simulink model "SWC_AFE_Control"  (R2022b)
settings: configuration reference "DC_DC_Charger_Configuration" (kept outside this file)
undefined symbols (not defined in the file or in its folder): DUTY_COUNT_LOWER_LMIT, DUTY_COUNT_UPPER_LMIT, Fault_Counts_perms, GRID_NORM_FREQ, GRID_VOLT_ADC_OFFSET, HALF_DUTY_PERIOD, INDUCTANCE, PI, PLL_FREQ_LOW_LIMIT, PLL_FREQ_UPP_LIMIT, PLL_PI_INTGRL_RESET, PLL_PI_KI, PLL_PI_KP, PLL_PI_LOWER_LIMIT, PLL_PI_UPPER_LIMIT, PLL_RATE, PLL_VD_ERROR_LIMIT, PLL_VD_ESTIMETED, PLL_VQ_ERROR_LIMIT, VDC_LOWER_LIM_SVPWM, VDC_UPPER_LIM_SVPWM
libraries: simulink x13, common_lib x8
(part 1 of 2)
settings Model: DataDictionary=SWC_Diag_AFE.sldd  ExtModeTrigDuration=8  Creator=E0654638  LastModifiedBy=E0660158
settings ConfigSetRef: SourceName=DC_DC_Charger_Configuration

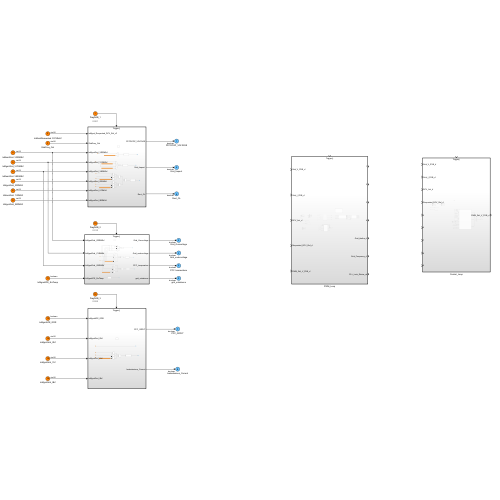
[thumbnail: Simulink's stored preview of the top-level diagram]
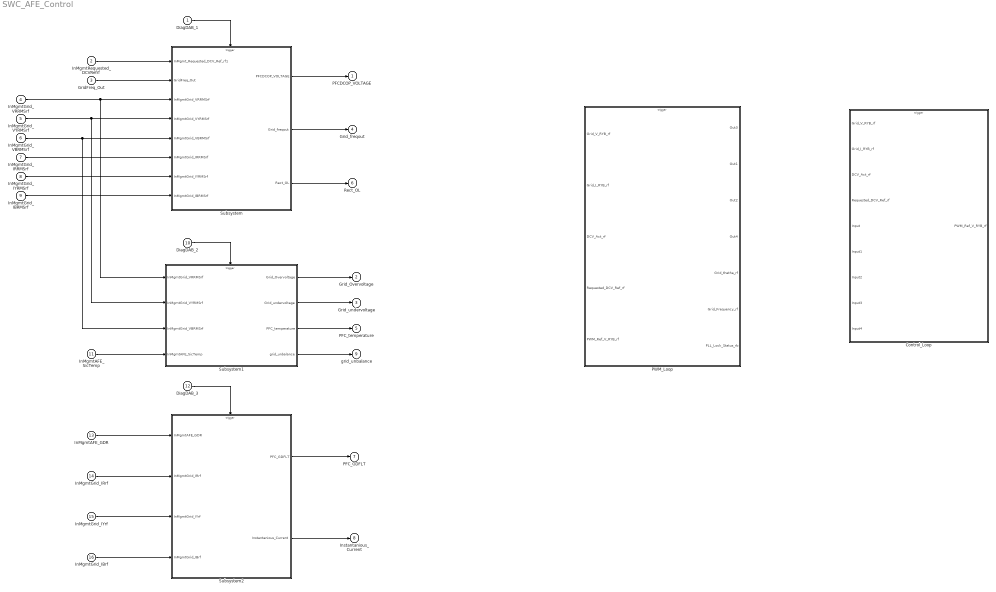
== system SWC_AFE_Control ==
  DiagDAB_1 : Inport  Description=Inverter HVDC voltage  OutMin=0  OutMax=1000  PortDimensions=1  SampleTime=0.001  OutputFunctionCall=on
      settings: AttributesFormatString=%<SampleTime>
  InMgmtRequested_DCVRefrf : Inport  Port=2  OutDataTypeStr=uint16
  GridFreq_Out : Inport  Port=3  OutDataTypeStr=uint16
  InMgmtGrid_VRRMSrf : Inport  Port=4  OutDataTypeStr=uint16
  InMgmtGrid_VYRMSrf : Inport  Port=5  OutDataTypeStr=uint16
  InMgmtGrid_VBRMSrf : Inport  Port=6  OutDataTypeStr=uint16
  InMgmtGrid_IRRMSrf : Inport  Port=7  OutDataTypeStr=uint16
  InMgmtGrid_IYRMSrf : Inport  Port=8  OutDataTypeStr=uint16
  InMgmtGrid_IBRMSrf : Inport  Port=9  OutDataTypeStr=uint16
  DiagDAB_2 : Inport  Description=Inverter HVDC voltage  Port=10  OutMin=0  OutMax=1000  PortDimensions=1  SampleTime=0.010  OutputFunctionCall=on
      settings: AttributesFormatString=%<SampleTime>
  InMgmtAFE_SicTemp : Inport  Port=11  OutDataTypeStr=boolean
  DiagDAB_3 : Inport  Description=Inverter HVDC voltage  Port=12  OutMin=0  OutMax=1000  PortDimensions=1  SampleTime=0.025  OutputFunctionCall=on
      settings: AttributesFormatString=%<SampleTime>
  InMgmtAFE_GDR : Inport  Port=13  OutDataTypeStr=boolean
  InMgmtGrid_IRrf : Inport  Port=14  OutDataTypeStr=uint16
  InMgmtGrid_IYrf : Inport  Port=15  OutDataTypeStr=uint16
  InMgmtGrid_IBrf : Inport  Port=16  OutDataTypeStr=uint16
  Control_Loop : Subsystem  Description=|  TreatAsAtomicUnit=on
      | @file      Control_Loop
      | @brief    All control related functions
      | @param[in]  required signals
      | @param[out] xxxxx
      | @return     None
      | @date       20/01/2023
      | @author     PKS (E0732241) @praveenksingh2@eaton.com
      | @copyright  Chief Engineer's office-EIIC
      settings: RTWSystemCode=Nonreusable function  RTWFcnNameOpts=Use subsystem name  RTWFileNameOpts=Use subsystem name
  PWM_Loop : Subsystem  Description=|  TreatAsAtomicUnit=on
      | @file       PWM_Loop
      | @brief      All algo related to PWM Control
      | @param[in]  required signals
      | @param[out] Duty values
      | @return     None
      | @date       20/01/2023
      | @author     PKS (E0732241) @praveenksingh2@eaton.com
      | @copyright  Chief Engineer's office-EIIC
      settings: RTWSystemCode=Nonreusable function  RTWFcnNameOpts=Use subsystem name  RTWFileNameOpts=Use subsystem name
  Subsystem : Subsystem
  Subsystem1 : Subsystem
  Subsystem2 : Subsystem
  PFCDCOP_VOLTAGE : Outport  OutDataTypeStr=boolean  VectorParamsAs1DForOutWhenUnconnected=off
  Grid_Overvoltage : Outport  Port=2  OutDataTypeStr=boolean  VectorParamsAs1DForOutWhenUnconnected=off
  Grid_undervoltage : Outport  Port=3  OutDataTypeStr=boolean  VectorParamsAs1DForOutWhenUnconnected=off
  "Grid_freqout " : Outport  Port=4  OutDataTypeStr=boolean  VectorParamsAs1DForOutWhenUnconnected=off
  PFC_temperature : Outport  Port=5  OutDataTypeStr=boolean  VectorParamsAs1DForOutWhenUnconnected=off
  Rect_OL : Outport  Port=6  OutDataTypeStr=boolean  VectorParamsAs1DForOutWhenUnconnected=off
  PFC_GDFLT : Outport  Port=7  OutDataTypeStr=boolean  VectorParamsAs1DForOutWhenUnconnected=off
  Instantanious_Current : Outport  Port=8  OutDataTypeStr=boolean  VectorParamsAs1DForOutWhenUnconnected=off
  grid_unbalance : Outport  Port=9  OutDataTypeStr=boolean  VectorParamsAs1DForOutWhenUnconnected=off
  wires:
  InMgmtRequested_DCVRefrf/1 -> Subsystem/1(InMgmt_Requested_DCV_Ref_rf1)
  Subsystem/1(PFCDCOP_VOLTAGE) -> PFCDCOP_VOLTAGE/1
  DiagDAB_1/1 -> Subsystem/Trigger
  InMgmtGrid_VRRMSrf/1 -> Subsystem1/1(InMgmtGrid_VRRMSrf), Subsystem/3(InMgmtGrid_VRRMSrf)
  InMgmtGrid_VYRMSrf/1 -> Subsystem1/2(InMgmtGrid_VYRMSrf), Subsystem/4(InMgmtGrid_VYRMSrf)
  InMgmtGrid_VBRMSrf/1 -> Subsystem1/3(InMgmtGrid_VBRMSrf), Subsystem/5(InMgmtGrid_VBRMSrf)
  Subsystem1/1(Grid_Overvoltage) -> Grid_Overvoltage/1
  DiagDAB_2/1 -> Subsystem1/Trigger
  Subsystem1/2(Grid_undervoltage) -> Grid_undervoltage/1
  GridFreq_Out/1 -> Subsystem/2(GridFreq_Out)
  Subsystem/2("Grid_freqout ") -> "Grid_freqout "/1
  InMgmtAFE_SicTemp/1 -> Subsystem1/4(InMgmtAFE_SicTemp)
  Subsystem1/3(PFC_temperature) -> PFC_temperature/1
  Subsystem/3(Rect_OL) -> Rect_OL/1
  Subsystem2/2(Instantanious_Current) -> Instantanious_Current/1
  InMgmtGrid_IBRMSrf/1 -> Subsystem/8(InMgmtGrid_IBRMSrf)
  InMgmtGrid_IYRMSrf/1 -> Subsystem/7(InMgmtGrid_IYRMSrf)
  InMgmtGrid_IRRMSrf/1 -> Subsystem/6(InMgmtGrid_IRRMSrf)
  DiagDAB_3/1 -> Subsystem2/Trigger
  Subsystem2/1(PFC_GDFLT) -> PFC_GDFLT/1
  InMgmtAFE_GDR/1 -> Subsystem2/1(InMgmtAFE_GDR)
  Subsystem1/4(grid_unbalance) -> grid_unbalance/1
  InMgmtGrid_IRrf/1 -> Subsystem2/2(InMgmtGrid_IRrf)
  InMgmtGrid_IYrf/1 -> Subsystem2/3(InMgmtGrid_IYrf)
  InMgmtGrid_IBrf/1 -> Subsystem2/4(InMgmtGrid_IBrf)

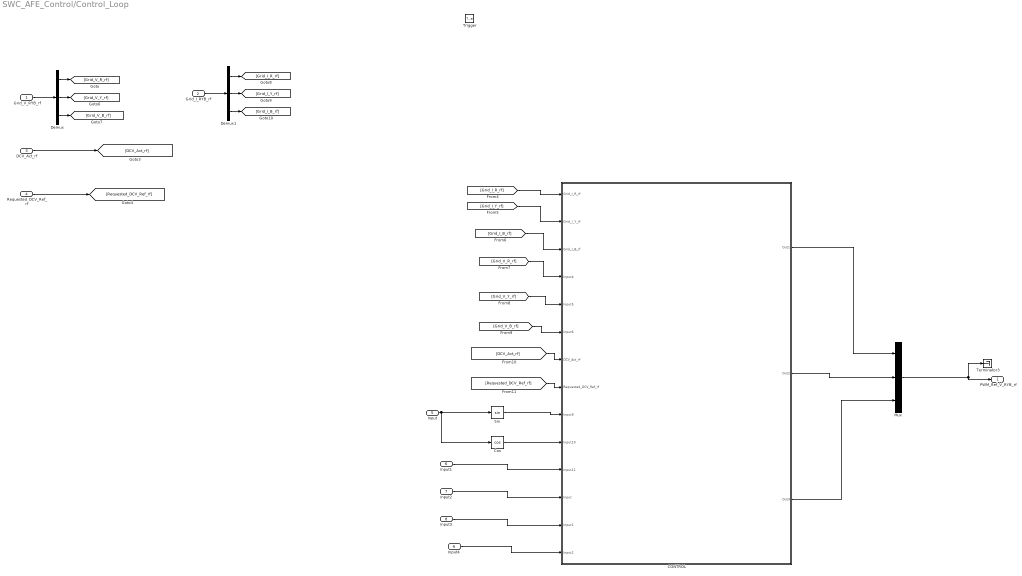
== system SWC_AFE_Control/Control_Loop ==
  Grid_V_RYB_rf : Inport
  Grid_I_RYB_rf : Inport  Port=2
  DCV_Act_rf : Inport  Port=3
  Requested_DCV_Ref_rf : Inport  Port=4
  Input : Inport  Port=5
  Input1 : Inport  Port=6
  Input2 : Inport  Port=7
  Input3 : Inport  Port=8
  Input4 : Inport  Port=9
  Trigger : TriggerPort  TriggerType=function-call  VariantControl=(inherit)
  CONTROL : Subsystem  Description=|  TreatAsAtomicUnit=on  RTWFcnName=PICntrllr2
      | @file      Control.c
      | @brief    All control related functions
      | @param[in]  required signals
      | @param[out] xxxxx
      | @return     None
      | @date       20/01/2023
      | @author     PKS (E0732241) @praveenksingh2@eaton.com
      | @copyright  Chief Engineer's office-EIIC
      settings: RTWFcnNameOpts=Use subsystem name  RTWFileNameOpts=Use subsystem name
  Cos : Trigonometry  Operator=cos
  Demux : Demux  Outputs=3
  Demux1 : Demux  Outputs=3
  Mux : Mux  Inputs=3
  Sin : Trigonometry
  Terminator3 : Terminator
  PWM_Ref_V_RYB_rf : Outport  OutDataTypeStr=single
  wires:
  Mux/1 -> Terminator3/1, PWM_Ref_V_RYB_rf/1
  Demux/1 -> [Grid_V_R_rf]
  Demux1/1 -> [Grid_I_R_rf]
  Demux/3 -> [Grid_V_B_rf]
  Grid_V_RYB_rf/1 -> Demux/1
  Demux1/2 -> [Grid_I_Y_rf]
  Demux1/3 -> [Grid_I_B_rf]
  Grid_I_RYB_rf/1 -> Demux1/1
  Demux/2 -> [Grid_V_Y_rf]
  Requested_DCV_Ref_rf/1 -> [Requested_DCV_Ref_rf]
  DCV_Act_rf/1 -> [DCV_Act_rf]
  [Grid_I_R_rf] -> CONTROL/1(Grid_I_R_rf)
  [Grid_I_Y_rf] -> CONTROL/2(Grid_I_Y_rf)
  [Grid_I_B_rf] -> CONTROL/3(Grid_I_B_rf)
  CONTROL/1(Out1) -> Mux/1
  CONTROL/2(Out2) -> Mux/2
  CONTROL/3(Out3) -> Mux/3
  [Grid_V_B_rf] -> CONTROL/6(Input6)
  [Grid_V_Y_rf] -> CONTROL/5(Input5)
  [Grid_V_R_rf] -> CONTROL/4(Input4)
  [DCV_Act_rf] -> CONTROL/7(DCV_Act_rf)
  [Requested_DCV_Ref_rf] -> CONTROL/8(Requested_DCV_Ref_rf)
  Input/1 -> Cos/1, Sin/1
  Sin/1 -> CONTROL/9(Input9)
  Cos/1 -> CONTROL/10(Input10)
  Input1/1 -> CONTROL/11(Input11)
  Input2/1 -> CONTROL/12(Input)
  Input3/1 -> CONTROL/13(Input1)
  Input4/1 -> CONTROL/14(Input2)

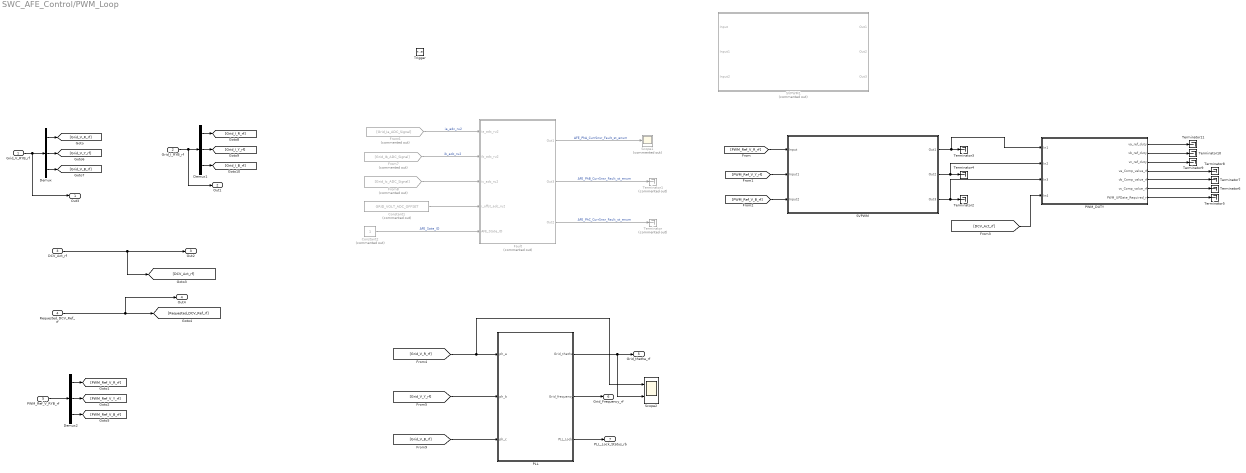
== system SWC_AFE_Control/PWM_Loop ==
  Grid_V_RYB_rf : Inport
  Grid_I_RYB_rf : Inport  Port=2
  DCV_Act_rf : Inport  Port=3
  Requested_DCV_Ref_rf : Inport  Port=4
  PWM_Ref_V_RYB_rf : Inport  Port=5
  Trigger : TriggerPort  TriggerType=function-call  VariantControl=(inherit)
  Constant1 : Constant  Commented=on  Value=GRID_VOLT_ADC_OFFSET
  Constant2 : Constant  Commented=on
  Demux : Demux  Outputs=3
  Demux1 : Demux  Outputs=3
  Demux2 : Demux  Outputs=3
  Fault : Subsystem  Description=|  Commented=on  TreatAsAtomicUnit=on  RTWFcnName=PICntrllr2
      | @file       Fault
      | @brief     All check related to protection and it imapct
      | @param[in]  required signals
      | @param[out] protection status and action taken
      | @return     None
      | @date       7/02/2023
      | @author     PKS (E0732241) @praveenksingh2@eaton.com
      | @copyright  Chief Engineer's office-EIIC
      settings: RTWSystemCode=Nonreusable function  RTWFcnNameOpts=Use subsystem name  RTWFileNameOpts=Use subsystem name
  From6 : From  Commented=on  GotoTag=Grid_Ia_ADC_Signal
  From7 : From  Commented=on  GotoTag=Grid_Ib_ADC_Signal
  From8 : From  Commented=on  GotoTag=Grid_Ic_ADC_Signal
  PLL : Subsystem  Description=|  TreatAsAtomicUnit=on  RTWFcnName=PICntrllr2
      | @file      pll.c
      | @brief      This is xxxx loop.
      | @param[in]  xxx
      | @param[out] yyyy
      | @return     None
      | @date       19/01/2023
      | @author     PKS E0732241
      | @copyright  Chief Engineer's office-EIIC
      settings: RTWFcnNameOpts=Use subsystem name  RTWFileNameOpts=Use subsystem name
  PWM_DUTY : Subsystem  TreatAsAtomicUnit=on
      settings: RTWFcnNameOpts=Use subsystem name  RTWFileNameOpts=Use subsystem name
  SVPWM : Subsystem  Description=|  TreatAsAtomicUnit=on  RTWFcnName=PICntrllr2
      | @file       svpwm.c
      | @brief      All algo related to PWM Control
      | @param[in]  required signals
      | @param[out] Duty values
      | @return     None
      | @date       20/01/2023
      | @author     PKS (E0732241) @praveenksingh2@eaton.com
      | @copyright  Chief Engineer's office-EIIC
      settings: RTWFcnNameOpts=Use subsystem name  RTWFileNameOpts=Use subsystem name
  SVPWM1 : Subsystem  Description=|  Commented=on  TreatAsAtomicUnit=on  RTWFcnName=PICntrllr2
      | @file       svpwm.c
      | @brief      All algo related to PWM Control
      | @param[in]  required signals
      | @param[out] Duty values
      | @return     None
      | @date       20/01/2023
      | @author     PKS (E0732241) @praveenksingh2@eaton.com
      | @copyright  Chief Engineer's office-EIIC
      settings: RTWFcnNameOpts=Use subsystem name  RTWFileNameOpts=Use subsystem name
  Scope1 : Scope  Commented=on
  Scope2 : Scope  NumInputPorts=2
  Terminator : Terminator  Commented=on
  Terminator1 : Terminator  Commented=on
  Terminator{2..11} (10 alike) : Terminator
  Out3 : Outport
  Out1 : Outport  Port=2
  Out2 : Outport  Port=3
  Out4 : Outport  Port=4
  Grid_thetha_rf : Outport  Port=5
  Grid_Frequency_rf : Outport  Port=6
  PLL_Lock_Status_rb : Outport  Port=7
  wires:
  Constant1/1 -> Fault/4(i_offst_adc_ru2)
  From8/1 -> Fault/3(ic_adc_ru2)
  From7/1 -> Fault/2(ib_adc_ru2)  "ib_adc_ru2"
  Constant2/1 -> Fault/5(AFE_State_ID)  "AFE_Sate_ID"
  From6/1 -> Fault/1(ia_adc_ru2)  "ia_adc_ru2"
  Fault/1(Out1) -> Scope1/1  "AFE_PhA_CurrSnsr_Fault_st_enum"
  Fault/3(Out2) -> Terminator/1  "AFE_PhC_CurrSnsr_Fault_st_enum"
  Fault/2(Out3) -> Terminator1/1  "AFE_PhB_CurrSnsr_Fault_st_enum"
  Requested_DCV_Ref_rf/1 -> Out4/1, [Requested_DCV_Ref_rf]
  DCV_Act_rf/1 -> Out2/1, [DCV_Act_rf]
  SVPWM/3(Out3) -> PWM_DUTY/3(In3), Terminator2/1
  SVPWM/2(Out2) -> PWM_DUTY/2(In2), Terminator4/1
  SVPWM/1(Out1) -> PWM_DUTY/1(In1), Terminator3/1
  Grid_V_RYB_rf/1 -> Out3/1, Demux/1
  Grid_I_RYB_rf/1 -> Out1/1, Demux1/1
  Demux/2 -> [Grid_V_Y_rf]
  Demux1/3 -> [Grid_I_B_rf]
  Demux/3 -> [Grid_V_B_rf]
  Demux1/1 -> [Grid_I_R_rf]
  Demux/1 -> [Grid_V_R_rf]
  Demux1/2 -> [Grid_I_Y_rf]
  Demux2/1 -> [PWM_Ref_V_R_rf]
  Demux2/3 -> [PWM_Ref_V_B_rf]
  PWM_Ref_V_RYB_rf/1 -> Demux2/1
  Demux2/2 -> [PWM_Ref_V_Y_rf]
  [PWM_Ref_V_R_rf] -> SVPWM/1(Input)
  [PWM_Ref_V_Y_rf] -> SVPWM/2(Input1)
  [PWM_Ref_V_B_rf] -> SVPWM/3(Input2)
  [Grid_V_R_rf] -> PLL/1(ph_a), Scope2/1
  [DCV_Act_rf] -> PWM_DUTY/4(In4)
  PWM_DUTY/7(PWM_UPDate_Required_rf) -> Terminator5/1
  PWM_DUTY/6(vc_Comp_value_rf) -> Terminator6/1
  PWM_DUTY/5(vb_Comp_value_rf) -> Terminator7/1
  PWM_DUTY/4(va_Comp_value_rf) -> Terminator8/1
  PWM_DUTY/3(vc_ref_duty) -> Terminator9/1
  PWM_DUTY/2(vb_ref_duty) -> Terminator10/1
  PWM_DUTY/1(va_ref_duty) -> Terminator11/1
  [Grid_V_Y_rf] -> PLL/2(ph_b)
  [Grid_V_B_rf] -> PLL/3(ph_c)
  PLL/3(PLL_Lock) -> PLL_Lock_Status_rb/1
  PLL/2(Grid_frequency) -> Grid_Frequency_rf/1
  PLL/1(Grid_thetha) -> Scope2/2, Grid_thetha_rf/1

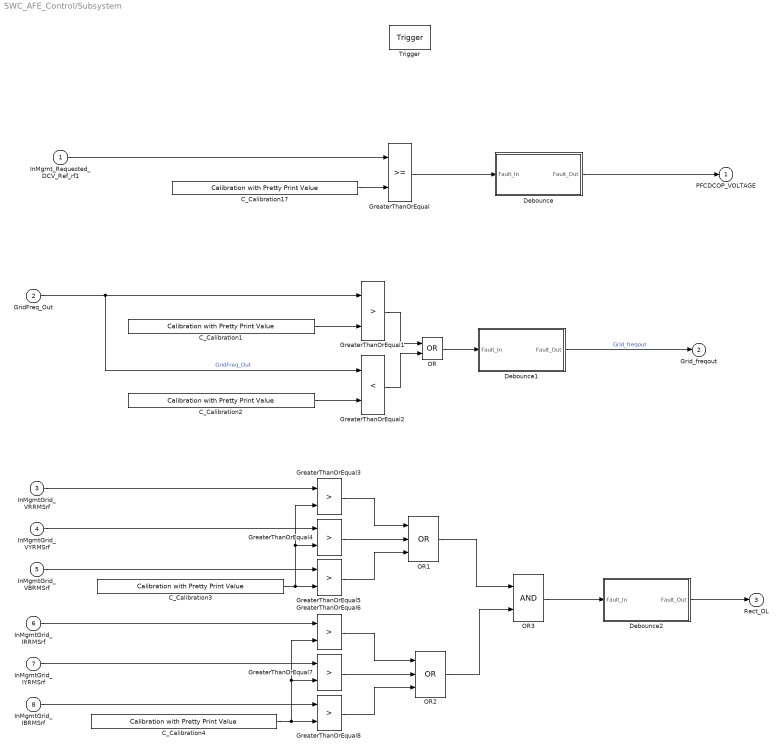
== system SWC_AFE_Control/Subsystem ==
  InMgmt_Requested_DCV_Ref_rf1 : Inport
  GridFreq_Out : Inport  Port=2
  InMgmtGrid_VRRMSrf : Inport  Port=3
  InMgmtGrid_VYRMSrf : Inport  Port=4
  InMgmtGrid_VBRMSrf : Inport  Port=5
  InMgmtGrid_IRRMSrf : Inport  Port=6
  InMgmtGrid_IYRMSrf : Inport  Port=7
  InMgmtGrid_IBRMSrf : Inport  Port=8
  Trigger : TriggerPort  TriggerType=function-call  VariantControl=(inherit)  SampleTime=-1  PortDimensions=1
  C_Calibration1 : common_lib/IO/Calibration with Pretty Print Value  CalValue=GridFreq_UThd  scaling=None
  C_Calibration17 : common_lib/IO/Calibration with Pretty Print Value  CalValue=InMgmtRequestedDCVRef_UThd  scaling=None
  C_Calibration2 : common_lib/IO/Calibration with Pretty Print Value  CalValue=GridFreq_LThd  scaling=None
  C_Calibration3 : common_lib/IO/Calibration with Pretty Print Value  CalValue=InMgmt_GridVRMS_LTHD  scaling=None
  C_Calibration4 : common_lib/IO/Calibration with Pretty Print Value  CalValue=InMgmt_GridIRMS_UTHD  scaling=None
  Debounce : Subsystem
  Debounce1 : Subsystem
  Debounce2 : Subsystem
  GreaterThanOrEqual : RelationalOperator  OutDataTypeStr=boolean  RndMeth=Simplest  InputSameDT=off
  GreaterThanOrEqual{1,3..8} (7 alike) : RelationalOperator  Operator=>  OutDataTypeStr=boolean  RndMeth=Simplest  InputSameDT=off
  GreaterThanOrEqual2 : RelationalOperator  Operator=<  OutDataTypeStr=boolean  RndMeth=Simplest  InputSameDT=off
  OR : Logic  Operator=OR  AllPortsSameDT=off  OutDataTypeStr=boolean
  OR1 : Logic  Operator=OR  Inputs=3  AllPortsSameDT=off  OutDataTypeStr=boolean
  OR2 : Logic  Operator=OR  Inputs=3  AllPortsSameDT=off  OutDataTypeStr=boolean
  OR3 : Logic  AllPortsSameDT=off  OutDataTypeStr=boolean
  PFCDCOP_VOLTAGE : Outport  VectorParamsAs1DForOutWhenUnconnected=off
  "Grid_freqout " : Outport  Port=2  VectorParamsAs1DForOutWhenUnconnected=off
  Rect_OL : Outport  Port=3  VectorParamsAs1DForOutWhenUnconnected=off
  wires:
  Debounce/1(Fault_Out) -> PFCDCOP_VOLTAGE/1
  C_Calibration17/1 -> GreaterThanOrEqual/2
  GreaterThanOrEqual/1 -> Debounce/1(Fault_In)
  InMgmt_Requested_DCV_Ref_rf1/1 -> GreaterThanOrEqual/1
  GridFreq_Out/1 -> GreaterThanOrEqual2/1, GreaterThanOrEqual1/1  "GridFreq_Out"
  C_Calibration1/1 -> GreaterThanOrEqual1/2
  C_Calibration2/1 -> GreaterThanOrEqual2/2
  GreaterThanOrEqual1/1 -> OR/1
  GreaterThanOrEqual2/1 -> OR/2
  OR/1 -> Debounce1/1(Fault_In)
  Debounce1/1(Fault_Out) -> "Grid_freqout "/1  "Grid_freqout"
  InMgmtGrid_VRRMSrf/1 -> GreaterThanOrEqual3/1
  InMgmtGrid_VYRMSrf/1 -> GreaterThanOrEqual4/1
  InMgmtGrid_VBRMSrf/1 -> GreaterThanOrEqual5/1
  C_Calibration3/1 -> GreaterThanOrEqual5/2, GreaterThanOrEqual4/2, GreaterThanOrEqual3/2
  InMgmtGrid_IRRMSrf/1 -> GreaterThanOrEqual6/1
  InMgmtGrid_IYRMSrf/1 -> GreaterThanOrEqual7/1
  InMgmtGrid_IBRMSrf/1 -> GreaterThanOrEqual8/1
  C_Calibration4/1 -> GreaterThanOrEqual7/2, GreaterThanOrEqual6/2, GreaterThanOrEqual8/2
  GreaterThanOrEqual3/1 -> OR1/1
  GreaterThanOrEqual4/1 -> OR1/2
  GreaterThanOrEqual5/1 -> OR1/3
  GreaterThanOrEqual7/1 -> OR2/2
  GreaterThanOrEqual6/1 -> OR2/1
  GreaterThanOrEqual8/1 -> OR2/3
  OR1/1 -> OR3/1
  OR2/1 -> OR3/2
  OR3/1 -> Debounce2/1(Fault_In)
  Debounce2/1(Fault_Out) -> Rect_OL/1

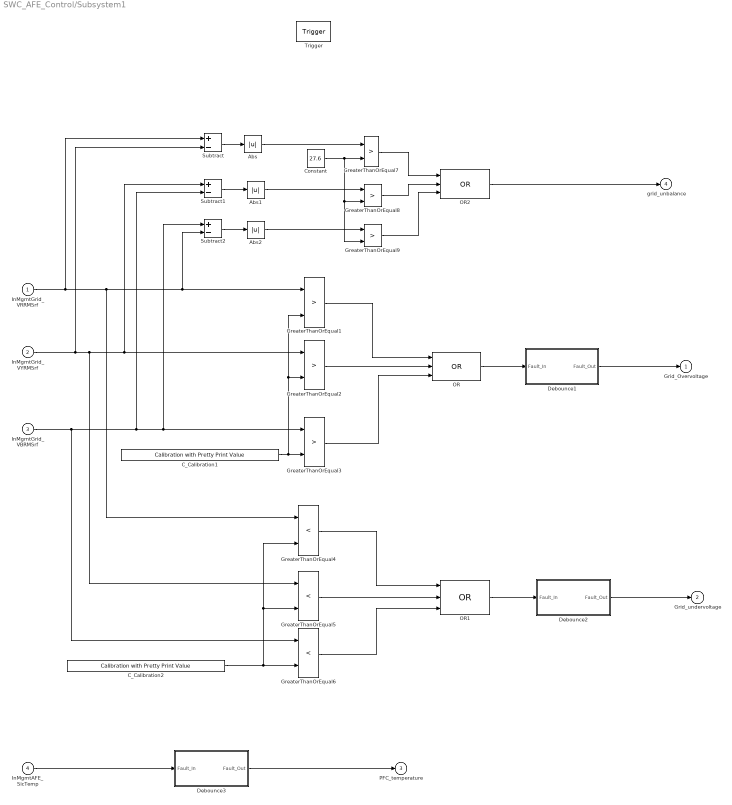
== system SWC_AFE_Control/Subsystem1 ==
  InMgmtGrid_VRRMSrf : Inport
  InMgmtGrid_VYRMSrf : Inport  Port=2
  InMgmtGrid_VBRMSrf : Inport  Port=3
  InMgmtAFE_SicTemp : Inport  Port=4
  Trigger : TriggerPort  TriggerType=function-call  VariantControl=(inherit)  SampleTime=-1  PortDimensions=1
  Abs : Abs  SaturateOnIntegerOverflow=off
  Abs1 : Abs  SaturateOnIntegerOverflow=off
  Abs2 : Abs  SaturateOnIntegerOverflow=off
  C_Calibration1 : common_lib/IO/Calibration with Pretty Print Value  CalValue=InMgmtGridVRYBRMS_UThd  scaling=None
  C_Calibration2 : common_lib/IO/Calibration with Pretty Print Value  CalValue=InMgmtGridVRYBRMS_LThd  scaling=None
  Constant : Constant  Value=27.6
  Debounce1 : Subsystem
  Debounce2 : Subsystem
  Debounce3 : Subsystem
  GreaterThanOrEqual{1..3,7..9} (6 alike) : RelationalOperator  Operator=>  OutDataTypeStr=boolean  RndMeth=Simplest  InputSameDT=off
  GreaterThanOrEqual4 : RelationalOperator  Operator=<  OutDataTypeStr=boolean  RndMeth=Simplest  InputSameDT=off
  GreaterThanOrEqual5 : RelationalOperator  Operator=<  OutDataTypeStr=boolean  RndMeth=Simplest  InputSameDT=off
  GreaterThanOrEqual6 : RelationalOperator  Operator=<  OutDataTypeStr=boolean  RndMeth=Simplest  InputSameDT=off
  OR : Logic  Operator=OR  Inputs=3  AllPortsSameDT=off  OutDataTypeStr=boolean
  OR1 : Logic  Operator=OR  Inputs=3  AllPortsSameDT=off  OutDataTypeStr=boolean
  OR2 : Logic  Operator=OR  Inputs=3  AllPortsSameDT=off  OutDataTypeStr=boolean
  Subtract : Sum  Inputs=+-
  Subtract1 : Sum  Inputs=+-
  Subtract2 : Sum  Inputs=+-
  Grid_Overvoltage : Outport  VectorParamsAs1DForOutWhenUnconnected=off
  Grid_undervoltage : Outport  Port=2  VectorParamsAs1DForOutWhenUnconnected=off
  PFC_temperature : Outport  Port=3  VectorParamsAs1DForOutWhenUnconnected=off
  grid_unbalance : Outport  Port=4  VectorParamsAs1DForOutWhenUnconnected=off
  wires:
  C_Calibration1/1 -> GreaterThanOrEqual1/2, GreaterThanOrEqual2/2, GreaterThanOrEqual3/2
  GreaterThanOrEqual2/1 -> OR/2
  GreaterThanOrEqual3/1 -> OR/3
  GreaterThanOrEqual1/1 -> OR/1
  InMgmtGrid_VRRMSrf/1 -> Subtract/1, GreaterThanOrEqual4/1, Subtract2/2, GreaterThanOrEqual1/1
  OR/1 -> Debounce1/1(Fault_In)
  InMgmtGrid_VYRMSrf/1 -> Subtract/2, GreaterThanOrEqual5/1, Subtract1/1, GreaterThanOrEqual2/1
  Debounce1/1(Fault_Out) -> Grid_Overvoltage/1
  InMgmtGrid_VBRMSrf/1 -> GreaterThanOrEqual6/1, Subtract1/2, Subtract2/1, GreaterThanOrEqual3/1
  C_Calibration2/1 -> GreaterThanOrEqual4/2, GreaterThanOrEqual5/2, GreaterThanOrEqual6/2
  GreaterThanOrEqual4/1 -> OR1/1
  GreaterThanOrEqual5/1 -> OR1/2
  GreaterThanOrEqual6/1 -> OR1/3
  OR1/1 -> Debounce2/1(Fault_In)
  Debounce2/1(Fault_Out) -> Grid_undervoltage/1
  InMgmtAFE_SicTemp/1 -> Debounce3/1(Fault_In)
  Debounce3/1(Fault_Out) -> PFC_temperature/1
  Subtract/1 -> Abs/1
  Constant/1 -> GreaterThanOrEqual9/2, GreaterThanOrEqual8/2, GreaterThanOrEqual7/2
  Abs/1 -> GreaterThanOrEqual7/1
  GreaterThanOrEqual7/1 -> OR2/1
  OR2/1 -> grid_unbalance/1
  Subtract1/1 -> Abs1/1
  Subtract2/1 -> Abs2/1
  Abs1/1 -> GreaterThanOrEqual8/1
  Abs2/1 -> GreaterThanOrEqual9/1
  GreaterThanOrEqual8/1 -> OR2/2
  GreaterThanOrEqual9/1 -> OR2/3

== system SWC_AFE_Control/Subsystem2 ==
  InMgmtAFE_GDR : Inport
  InMgmtGrid_IRrf : Inport  Port=2
  InMgmtGrid_IYrf : Inport  Port=3
  InMgmtGrid_IBrf : Inport  Port=4
  Trigger : TriggerPort  TriggerType=function-call  VariantControl=(inherit)  SampleTime=-1  PortDimensions=1
  C_Calibration4 : common_lib/IO/Calibration with Pretty Print Value  CalValue=InMgmtGridI_UTHD  scaling=None
  Debounce2 : Subsystem
  GreaterThanOrEqual6 : RelationalOperator  OutDataTypeStr=boolean  RndMeth=Simplest  InputSameDT=off
  GreaterThanOrEqual7 : RelationalOperator  OutDataTypeStr=boolean  RndMeth=Simplest  InputSameDT=off
  GreaterThanOrEqual8 : RelationalOperator  OutDataTypeStr=boolean  RndMeth=Simplest  InputSameDT=off
  OR2 : Logic  Operator=OR  Inputs=3  AllPortsSameDT=off  OutDataTypeStr=boolean
  PFC_GDFLT : Outport  VectorParamsAs1DForOutWhenUnconnected=off
  Instantanious_Current : Outport  Port=2  VectorParamsAs1DForOutWhenUnconnected=off
  wires:
  Debounce2/1(Fault_Out) -> Instantanious_Current/1
  OR2/1 -> Debounce2/1(Fault_In)
  GreaterThanOrEqual8/1 -> OR2/3
  GreaterThanOrEqual6/1 -> OR2/1
  GreaterThanOrEqual7/1 -> OR2/2
  C_Calibration4/1 -> GreaterThanOrEqual8/2, GreaterThanOrEqual6/2, GreaterThanOrEqual7/2
  InMgmtGrid_IBrf/1 -> GreaterThanOrEqual8/1
  InMgmtGrid_IYrf/1 -> GreaterThanOrEqual7/1
  InMgmtGrid_IRrf/1 -> GreaterThanOrEqual6/1
  InMgmtAFE_GDR/1 -> PFC_GDFLT/1

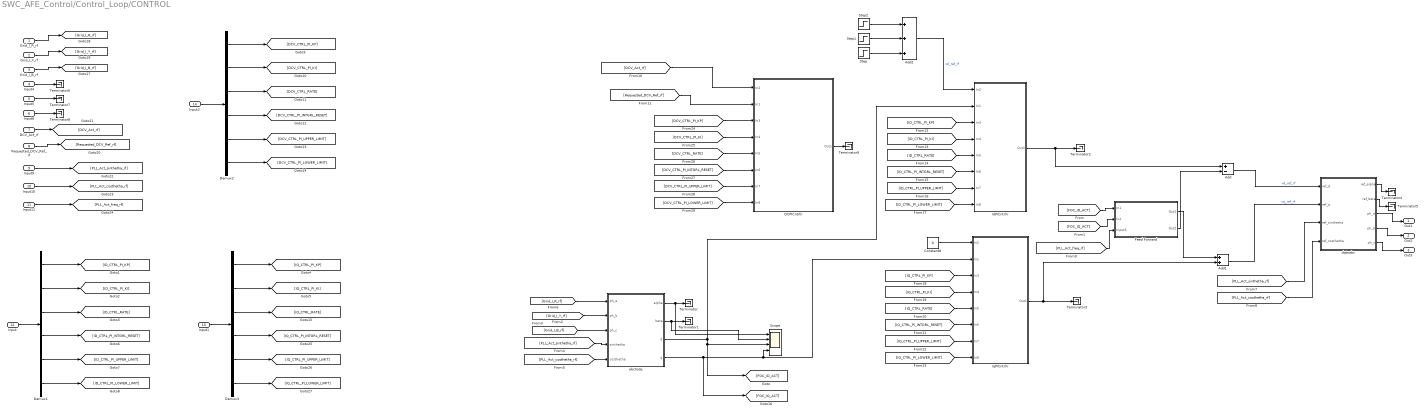
== system SWC_AFE_Control/Control_Loop/CONTROL ==
  Grid_I_R_rf : Inport
  Grid_I_Y_rf : Inport  Port=2
  Grid_I_B_rf : Inport  Port=3
  Input4 : Inport  Port=4
  Input5 : Inport  Port=5
  Input6 : Inport  Port=6
  DCV_Act_rf : Inport  Port=7
  Requested_DCV_Ref_rf : Inport  Port=8
  Input9 : Inport  Port=9
  Input10 : Inport  Port=10
  Input11 : Inport  Port=11
  Input : Inport  Port=12
  Input1 : Inport  Port=13
  Input2 : Inport  Port=14
  Add : Sum  Inputs=+-
  Add1 : Sum
  Add2 : Sum  Inputs=+++
  Constant8 : Constant  Value=0  SampleTime=-1
  DCPICntrllr : Subsystem  Description=|  TreatAsAtomicUnit=on  RTWFcnName=PICntrllr2
      | @file       DCPICntrllr.c
      | @brief      This is PI Controll loop.
      | @param[in]  xxx
      | @param[out] yyyy
      | @return     None
      | @date       19/01/2023
      | @author     PKS E0732241
      | @copyright  Chief Engineer's office-EIIC
      settings: RTWFcnNameOpts=Use subsystem name  RTWFileNameOpts=Use subsystem name
  Demux1 : Demux  Outputs=6
  Demux2 : Demux  Outputs=6
  Demux3 : Demux  Outputs=6
  Feed Forward : Subsystem
  IdPICntrllr : Subsystem  Description=|  TreatAsAtomicUnit=on  RTWFcnName=PICntrllr2
      | @file       IdPICntrllr.c
      | @brief      This is PI Controll loop.
      | @param[in]  xxx
      | @param[out] yyyy
      | @return     None
      | @date       19/01/2023
      | @author     PKS E0732241
      | @copyright  Chief Engineer's office-EIIC
      settings: RTWFcnNameOpts=Use subsystem name  RTWFileNameOpts=Use subsystem name
  IqPICntrllr : Subsystem  Description=|  TreatAsAtomicUnit=on  RTWFcnName=PICntrllr2
      | @file       IqPICntrllr.c
      | @brief      This is PI Controll loop.
      | @param[in]  xxx
      | @param[out] yyyy
      | @return     None
      | @date       19/01/2023
      | @author     PKS E0732241
      | @copyright  Chief Engineer's office-EIIC
      settings: RTWFcnNameOpts=Use subsystem name  RTWFileNameOpts=Use subsystem name
  Scope : Scope  NumInputPorts=4
  Step : Step  Time=0.5  After=14
  Step1 : Step  Time=1.0  After=14
  Step2 : Step  Time=1.5  After=14
  Terminator{,1..9} (10 alike) : Terminator
  abctodq : Subsystem  Description=|  TreatAsAtomicUnit=on  RTWFcnName=PICntrllr2
      | @file       abctodq.c
      | @brief      This is abctodq loop.
      | @param[in]  xxx
      | @param[out] yyyy
      | @return     None
      | @date       19/01/2023
      | @author     PKS E0732241
      | @copyright  Chief Engineer's office-EIIC
      settings: RTWFcnNameOpts=Use subsystem name  RTWFileNameOpts=Use subsystem name
  dqtoabc : Subsystem  Description=|  TreatAsAtomicUnit=on  RTWFcnName=PICntrllr2
      | @file       DQTOABC.c
      | @brief      This is dqtoabc loop.
      | @param[in]  xxx
      | @param[out] yyyy
      | @return     None
      | @date       19/01/2023
      | @author     PKS E0732241
      | @copyright  Chief Engineer's office-EIIC
      settings: RTWFcnNameOpts=Use subsystem name  RTWFileNameOpts=Use subsystem name
  Out1 : Outport
  Out2 : Outport  Port=2
  Out3 : Outport  Port=3
  wires:
  Demux1/2 -> [ID_CTRL_PI_KI]
  Demux1/1 -> [ID_CTRL_PI_KP]
  Input/1 -> Demux1/1
  Demux1/3 -> [ID_CTRL_RATE]
  Demux1/4 -> [ID_CTRL_PI_INTGRL_RESET]
  Demux1/5 -> [ID_CTRL_PI_UPPER_LIMIT]
  Demux1/6 -> [ID_CTRL_PI_LOWER_LIMIT]
  Demux2/4 -> [DCV_CTRL_PI_INTGRL_RESET]
  Demux2/5 -> [DCV_CTRL_PI_UPPER_LIMIT]
  Input2/1 -> Demux2/1
  Demux2/1 -> [DCV_CTRL_PI_KP]
  Demux2/2 -> [DCV_CTRL_PI_KI]
  Demux2/3 -> [DCV_CTRL_RATE]
  Demux2/6 -> [DCV_CTRL_PI_LOWER_LIMIT]
  abctodq/1(alpha) -> Scope/1, Terminator/1
  IqPICntrllr/1(Out1) -> Add1/2, Terminator3/1
  IdPICntrllr/1(Out1) -> Add/1, Terminator2/1
  dqtoabc/3(ph_a) -> Out1/1
  dqtoabc/5(ph_c) -> Out3/1
  Feed Forward/2(Out2) -> Add/2
  dqtoabc/4(ph_b) -> Out2/1
  [Requested_DCV_Ref_rf] -> DCPICntrllr/2(In1)
  [ID_CTRL_PI_INTGRL_RESET] -> IdPICntrllr/6(In6)
  [FOC_IQ_ACT] -> Feed Forward/2(In2)
  [IQ_CTRL_PI_INTGRL_RESET] -> IqPICntrllr/6(In6)
  [IQ_CTRL_RATE] -> IqPICntrllr/5(In5)
  [ID_CTRL_PI_KP] -> IdPICntrllr/3(In3)
  [IQ_CTRL_PI_KI] -> IqPICntrllr/4(In4)
  [ID_CTRL_RATE] -> IdPICntrllr/5(In5)
  [ID_CTRL_PI_KI] -> IdPICntrllr/4(In4)
  Constant8/1 -> IqPICntrllr/1(In2)
  [ID_CTRL_PI_LOWER_LIMIT] -> IdPICntrllr/8(In8)
  [IQ_CTRL_PI_LOWER_LIMIT] -> IqPICntrllr/8(In8)
  [DCV_Act_rf] -> DCPICntrllr/1(In2)
  [DCV_CTRL_PI_UPPER_LIMIT] -> DCPICntrllr/7(In7)
  [FOC_ID_ACT] -> Feed Forward/1(In1)
  [DCV_CTRL_PI_LOWER_LIMIT] -> DCPICntrllr/8(In8)
  [DCV_CTRL_PI_KP] -> DCPICntrllr/3(In3)
  [DCV_CTRL_PI_INTGRL_RESET] -> DCPICntrllr/6(In6)
  [DCV_CTRL_RATE] -> DCPICntrllr/5(In5)
  [DCV_CTRL_PI_KI] -> DCPICntrllr/4(In4)
  Feed Forward/1(Out1) -> Add1/1
  abctodq/4(q) -> [FOC_IQ_ACT], IqPICntrllr/2(In1), Scope/4
  abctodq/2(beta) -> Scope/2, Terminator1/1
  [IQ_CTRL_PI_KP] -> IqPICntrllr/3(In3)
  Add1/1 -> dqtoabc/2(ref_q)  "vq_ref_rf"
  dqtoabc/1(ref_alpha) -> Terminator4/1
  Add/1 -> dqtoabc/1(ref_d)  "vd_ref_rf"
  dqtoabc/2(ref_beta) -> Terminator5/1
  [ID_CTRL_PI_UPPER_LIMIT] -> IdPICntrllr/7(In7)
  abctodq/3(d) -> [FOC_ID_ACT], Scope/3, IdPICntrllr/2(In1)
  [IQ_CTRL_PI_UPPER_LIMIT] -> IqPICntrllr/7(In7)
  Input6/1 -> Terminator8/1
  Input5/1 -> Terminator7/1
  Input4/1 -> Terminator6/1
  Grid_I_B_rf/1 -> [Grid_I_B_rf]
  Grid_I_Y_rf/1 -> [Grid_I_Y_rf]
  Grid_I_R_rf/1 -> [Grid_I_R_rf]
  [Grid_I_R_rf] -> abctodq/1(ph_a)
  [Grid_I_Y_rf] -> abctodq/2(ph_b)
  [Grid_I_B_rf] -> abctodq/3(ph_c)
  Requested_DCV_Ref_rf/1 -> [Requested_DCV_Ref_rf]
  DCV_Act_rf/1 -> [DCV_Act_rf]
  Input9/1 -> [PLL_Act_sinthetha_rf]
  Input10/1 -> [PLL_Act_costhetha_rf]
  [PLL_Act_sinthetha_rf] -> abctodq/4(sinthetha)
  [PLL_Act_costhetha_rf] -> abctodq/5(costhetha)
  [PLL_Act_sinthetha_rf] -> dqtoabc/3(ref_sinthetha)
  [PLL_Act_costhetha_rf] -> dqtoabc/4(ref_costhetha)
  Input11/1 -> [PLL_Act_freq_rf]
  [PLL_Act_freq_rf] -> Feed Forward/3(Input5)
  Input1/1 -> Demux3/1
  Demux3/2 -> [IQ_CTRL_PI_KI]
  Demux3/3 -> [IQ_CTRL_RATE]
  Demux3/6 -> [IQ_CTRL_PI_LOWER_LIMIT]
  Demux3/1 -> [IQ_CTRL_PI_KP]
  Demux3/5 -> [IQ_CTRL_PI_UPPER_LIMIT]
  Demux3/4 -> [IQ_CTRL_PI_INTGRL_RESET]
  DCPICntrllr/1(Out1) -> Terminator9/1
  Add2/1 -> IdPICntrllr/1(In2)  "vd_ref_rf"
  Step/1 -> Add2/3
  Step1/1 -> Add2/2
  Step2/1 -> Add2/1

== system SWC_AFE_Control/PWM_Loop/Fault ==
  ia_adc_ru2 : Inport
  ib_adc_ru2 : Inport  Port=2
  ic_adc_ru2 : Inport  Port=3
  i_offst_adc_ru2 : Inport  Port=4
  AFE_State_ID : Inport  Port=5
  CurrentFaults : Subsystem
  Out1 : Outport
  Out3 : Outport  Port=2
  Out2 : Outport  Port=3
  wires:
  ia_adc_ru2/1 -> CurrentFaults/1(Ia_adc_ru2)  "ia_adc_ru2"
  ib_adc_ru2/1 -> CurrentFaults/2(Ib_adc_ru2)  "ib_adc_ru2"
  ic_adc_ru2/1 -> CurrentFaults/3(Ic_adc_ru2)  "ic_adc_ru2"
  i_offst_adc_ru2/1 -> CurrentFaults/4(Iabc_offset_ru2)  "i_offst_adc_ru2"
  AFE_State_ID/1 -> CurrentFaults/5(AFE_State_ID)  "AFE_State_ID"
  CurrentFaults/1(Out1) -> Out1/1  "AFE_PhA_CurrSnsr_Fault_st_enum"
  CurrentFaults/2(Out2) -> Out2/1  "AFE_PhB_CurrSnsr_Fault_st_enum"
  CurrentFaults/3(Out3) -> Out3/1  "AFE_PhC_CurrSnsr_Fault_st_enum"

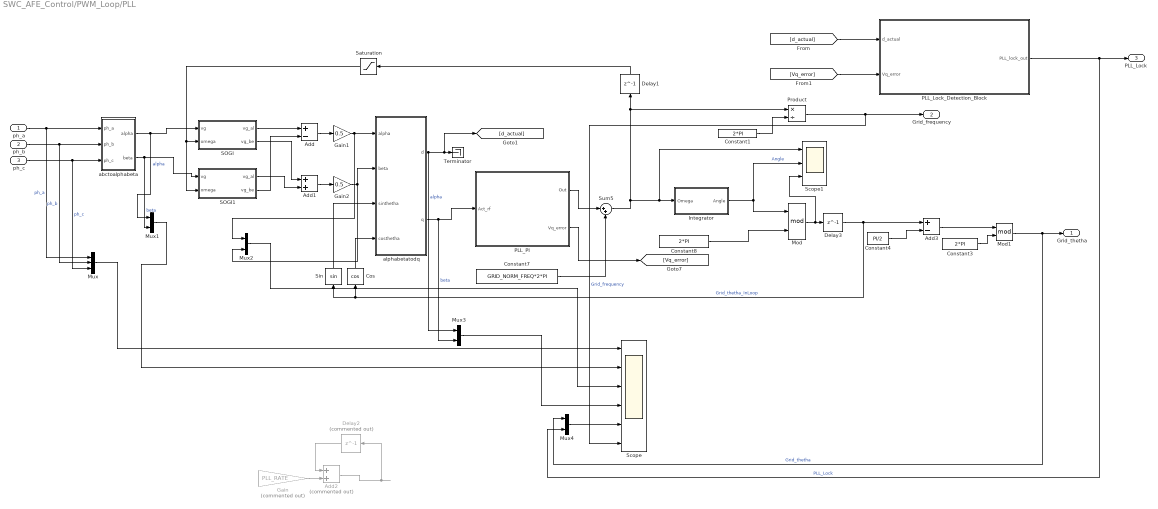
== system SWC_AFE_Control/PWM_Loop/PLL ==
  ph_a : Inport
  ph_b : Inport  Port=2
  ph_c : Inport  Port=3
  Add : Sum  Inputs=+-
  Add1 : Sum
  Add2 : Sum  Commented=on  OutDataTypeStr=single
  Add3 : Sum  Inputs=+-  OutDataTypeStr=single
  Constant1 : Constant  Value=2*PI  OutDataTypeStr=single  SampleTime=-1
  Constant3 : Constant  Value=2*PI  OutDataTypeStr=single  SampleTime=-1
  Constant4 : Constant  Value=PI/2  OutDataTypeStr=single  SampleTime=-1
  Constant7 : Constant  Value=GRID_NORM_FREQ*2*PI  SampleTime=-1
  Constant8 : Constant  Value=2*PI  OutDataTypeStr=single  SampleTime=-1
  Cos : Trigonometry  Operator=cos
  Delay1 : Delay  DelayLength=1
  Delay2 : Delay  Commented=on  DelayLength=1
  Delay3 : Delay  DelayLength=1
  Gain : Gain  Commented=on  Gain=PLL_RATE
  Gain1 : Gain  Gain=0.5
  Gain2 : Gain  Gain=0.5
  Integrator : Subsystem
  Mod : Math  Operator=mod
  Mod1 : Math  Operator=mod
  Mux : Mux  Inputs=3
  Mux{1..4} (4 alike) : Mux  Inputs=2
  PLL_Lock_Detection_Block : Subsystem
  PLL_PI : Subsystem
  Product : Product  Inputs=*/  OutDataTypeStr=single
  SOGI : Subsystem
  SOGI1 : Subsystem
  Saturation : Saturate  UpperLimit=PLL_FREQ_UPP_LIMIT  LowerLimit=PLL_FREQ_LOW_LIMIT
  Scope : Scope  NumInputPorts=6
  Scope1 : Scope  NumInputPorts=3
  Sin : Trigonometry
  Sum5 : Sum  Inputs=|++
  Terminator : Terminator
  abctoalphabeta : Subsystem  TreatAsAtomicUnit=on
  alphabetatodq : Subsystem
  Grid_thetha : Outport  OutDataTypeStr=single
  Grid_frequency : Outport  Port=2  OutDataTypeStr=single
  PLL_Lock : Outport  Port=3  OutDataTypeStr=single
  wires:
  Mux4/1 -> Scope/5
  PLL_PI/2(Vq_error) -> [Vq_error]
  [Vq_error] -> PLL_Lock_Detection_Block/2(Vq_error)
  PLL_Lock_Detection_Block/1(PLL_lock_out) -> PLL_Lock/1, Mux4/2  "PLL_Lock"
  [d_actual] -> PLL_Lock_Detection_Block/1(d_actual)
  Saturation/1 -> SOGI/2(omega), SOGI1/2(omega)
  Constant4/1 -> Add3/2
  Constant3/1 -> Mod1/2
  Mod1/1 -> Grid_thetha/1, Mux4/1  "Grid_thetha"
  Add3/1 -> Mod1/1
  Constant8/1 -> Mod/2
  Mux3/1 -> Scope/4
  Mux2/1 -> Scope/3
  Mux1/1 -> Scope/2
  alphabetatodq/2(q) -> PLL_PI/1(Act_rf), Mux3/2  "beta"
  alphabetatodq/1(d) -> Terminator/1, [d_actual], Mux3/1  "alpha"
  Mux/1 -> Scope/1
  Gain2/1 -> Mux2/2, alphabetatodq/2(beta)
  Gain1/1 -> alphabetatodq/1(alpha), Mux2/1
  SOGI1/1(vg_al) -> Add1/2
  SOGI/2(vg_be) -> Add1/1
  SOGI1/2(vg_be) -> Add/2
  Constant1/1 -> Product/2
  Product/1 -> Grid_frequency/1, Scope/6  "Grid_frequency"
  Sum5/1 -> Product/1, Delay1/1, Scope1/1, Integrator/1(Omega)
  Constant7/1 -> Sum5/2
  PLL_PI/1(Out) -> Sum5/1
  Sin/1 -> alphabetatodq/3(sinthetha)
  Cos/1 -> alphabetatodq/4(costhetha)
  Delay3/1 -> Cos/1, Sin/1, Add3/1  "Grid_thetha_InLoop"
  Mod/1 -> Scope1/3, Delay3/1
  Add1/1 -> Gain2/1
  Add/1 -> Gain1/1
  SOGI/1(vg_al) -> Add/1
  abctoalphabeta/2(beta) -> Mux1/2, SOGI1/1(vg)  "beta"
  abctoalphabeta/1(alpha) -> SOGI/1(vg), Mux1/1  "alpha"
  ph_a/1 -> abctoalphabeta/1(ph_a), Mux/1  "ph_a"
  ph_b/1 -> abctoalphabeta/2(ph_b), Mux/2  "ph_b"
  ph_c/1 -> abctoalphabeta/3(ph_c), Mux/3  "ph_c"
  Add2/1 -> Delay2/1
  Gain/1 -> Add2/2
  ? -> Gain/1
  Delay2/1 -> Add2/1
  Delay1/1 -> Saturation/1
  Integrator/1(Angle) -> Scope1/2, Mod/1  "Angle"

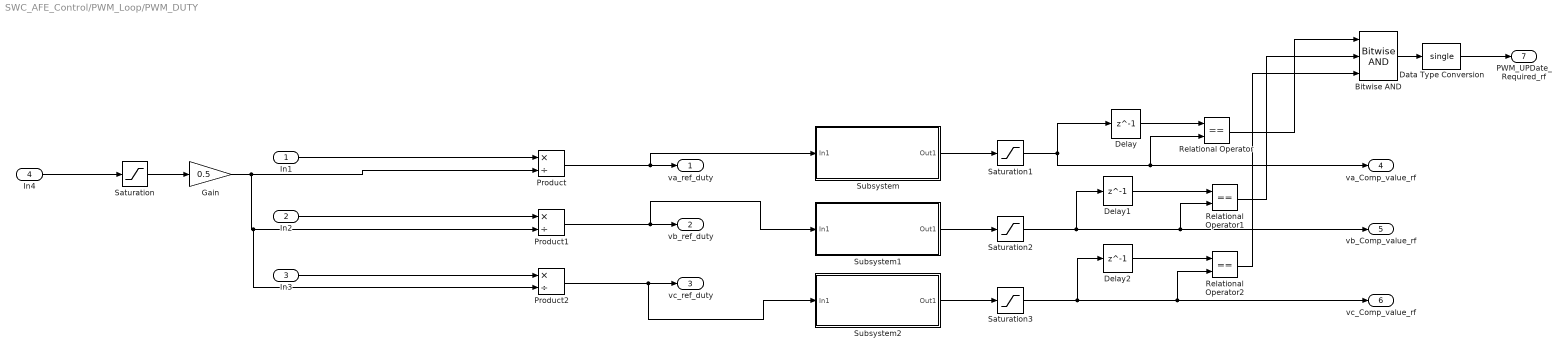
== system SWC_AFE_Control/PWM_Loop/PWM_DUTY ==
  In1 : Inport
  In2 : Inport  Port=2
  In3 : Inport  Port=3
  In4 : Inport  Port=4
  Bitwise AND : simulink/Logic and Bit Operations/Bitwise Operator  logicop=AND  UseBitMask=off  NumInputPorts=3  BitMask=bin2dec('11011001')  BitMaskRealWorld=Stored Integer
      settings: LibrarySourceBlock=|
      | simulink/Quick Insert/Logic and Bit
      | Operations/Bitwise AND
  Data Type Conversion : DataTypeConversion  OutDataTypeStr=single  SaturateOnIntegerOverflow=off  RndMeth=Floor
  Delay : Delay  DelayLength=1
  Delay1 : Delay  DelayLength=1
  Delay2 : Delay  DelayLength=1
  Gain : Gain  Gain=0.5
  Product : Product  Inputs=*/
  Product1 : Product  Inputs=*/
  Product2 : Product  Inputs=*/
  Relational Operator : RelationalOperator  Operator===  OutDataTypeStr=boolean  RndMeth=Simplest  InputSameDT=off
  Relational Operator1 : RelationalOperator  Operator===  OutDataTypeStr=boolean  RndMeth=Simplest  InputSameDT=off
  Relational Operator2 : RelationalOperator  Operator===  OutDataTypeStr=boolean  RndMeth=Simplest  InputSameDT=off
  Saturation : Saturate  UpperLimit=VDC_UPPER_LIM_SVPWM  LowerLimit=VDC_LOWER_LIM_SVPWM
  Saturation1 : Saturate  UpperLimit=DUTY_COUNT_UPPER_LMIT  LowerLimit=DUTY_COUNT_LOWER_LMIT
  Saturation2 : Saturate  UpperLimit=DUTY_COUNT_UPPER_LMIT  LowerLimit=DUTY_COUNT_LOWER_LMIT
  Saturation3 : Saturate  UpperLimit=DUTY_COUNT_UPPER_LMIT  LowerLimit=DUTY_COUNT_LOWER_LMIT
  Subsystem : Subsystem
  Subsystem1 : Subsystem
  Subsystem2 : Subsystem
  va_ref_duty : Outport
  vb_ref_duty : Outport  Port=2
  vc_ref_duty : Outport  Port=3
  va_Comp_value_rf : Outport  Port=4  OutDataTypeStr=single
  vb_Comp_value_rf : Outport  Port=5  OutDataTypeStr=single
  vc_Comp_value_rf : Outport  Port=6  OutDataTypeStr=single
  PWM_UPDate_Required_rf : Outport  Port=7  OutDataTypeStr=single
  wires:
  Saturation/1 -> Gain/1
  In4/1 -> Saturation/1
  Product/1 -> Subsystem/1(In1), va_ref_duty/1
  In1/1 -> Product/1
  In2/1 -> Product1/1
  In3/1 -> Product2/1
  Gain/1 -> Product2/2, Product1/2, Product/2
  Subsystem/1(Out1) -> Saturation1/1
  Subsystem1/1(Out1) -> Saturation2/1
  Product1/1 -> Subsystem1/1(In1), vb_ref_duty/1
  Product2/1 -> vc_ref_duty/1, Subsystem2/1(In1)
  Saturation1/1 -> Relational Operator/2, va_Comp_value_rf/1, Delay/1
  Saturation2/1 -> Relational Operator1/2, vb_Comp_value_rf/1, Delay1/1
  Subsystem2/1(Out1) -> Saturation3/1
  Saturation3/1 -> Delay2/1, Relational Operator2/2, vc_Comp_value_rf/1
  Delay/1 -> Relational Operator/1
  Delay1/1 -> Relational Operator1/1
  Delay2/1 -> Relational Operator2/1
  Relational Operator/1 -> Bitwise AND/1
  Relational Operator1/1 -> Bitwise AND/2
  Relational Operator2/1 -> Bitwise AND/3
  Bitwise AND/1 -> Data Type Conversion/1
  Data Type Conversion/1 -> PWM_UPDate_Required_rf/1

== system SWC_AFE_Control/PWM_Loop/SVPWM ==
  note: Carrier Based Space Vector Modulation based on common mode voltage addition
  Input : Inport
  Input1 : Inport  Port=2
  Input2 : Inport  Port=3
  Add : Sum
  Add1 : Sum  Inputs=+-
  Demux : Demux  Outputs=3
  Gain : Gain  Gain=0.5
  Min : MinMax
  Min1 : MinMax  Function=max
  Mux : Mux  Inputs=3
  Out1 : Outport
  Out2 : Outport  Port=2
  Out3 : Outport  Port=3
  wires:
  Add/1 -> Gain/1
  Min1/1 -> Add/2
  Min/1 -> Add/1
  Input/1 -> Mux/1  "va_ref"
  Input1/1 -> Mux/2  "vb_ref"
  Input2/1 -> Mux/3  "vc_ref"
  Mux/1 -> Add1/1, Min1/1, Min/1
  Add1/1 -> Demux/1
  Demux/1 -> Out1/1
  Demux/2 -> Out2/1
  Demux/3 -> Out3/1
  Gain/1 -> Add1/2

== system SWC_AFE_Control/PWM_Loop/SVPWM1 ==
  note: Carrier Based Space Vector Modulation based on common mode voltage addition
  Input : Inport
  Input1 : Inport  Port=2
  Input2 : Inport  Port=3
  Add : Sum
  Add1 : Sum  Inputs=+-
  Add2 : Sum  Inputs=+-
  Add3 : Sum  Inputs=+-
  Gain : Gain  Gain=0.5
  Min : MinMax  Inputs=3
  Min1 : MinMax  Function=max  Inputs=3
  Out1 : Outport
  Out2 : Outport  Port=2
  Out3 : Outport  Port=3
  wires:
  Input/1 -> Min/1, Min1/1, Add1/1  "va_ref"
  Input2/1 -> Min/3, Min1/3, Add3/1  "vc_ref"
  Min/1 -> Add/1
  Min1/1 -> Add/2
  Add/1 -> Gain/1
  Gain/1 -> Add1/2, Add2/2, Add3/2
  Add2/1 -> Out2/1
  Input1/1 -> Min/2, Min1/2, Add2/1  "vb_ref"
  Add1/1 -> Out1/1
  Add3/1 -> Out3/1

== system SWC_AFE_Control/Subsystem/Debounce ==
  Fault_In : Inport
  Add : Sum
  Delay1 : Delay  DelayLength=1
  Product : Product
  Saturation : Saturate  UpperLimit=(1*20)+1  LowerLimit=0
  Switch : Switch  Threshold=(1*20)  SaturateOnIntegerOverflow=off  InputSameDT=off
  and : Logic  AllPortsSameDT=off  OutDataTypeStr=boolean
  one : Constant
  zero : Constant  Value=0
  Fault_Out : Outport  VectorParamsAs1DForOutWhenUnconnected=off
  wires:
  Fault_In/1 -> Add/1, Product/1, and/2
  Product/1 -> Delay1/1
  Saturation/1 -> Switch/2, Product/2
  Add/1 -> Saturation/1
  zero/1 -> Switch/3
  one/1 -> Switch/1
  Delay1/1 -> Add/2
  Switch/1 -> and/1
  and/1 -> Fault_Out/1

== system SWC_AFE_Control/Subsystem/Debounce1 ==
  Fault_In : Inport
  Add : Sum
  Delay1 : Delay  DelayLength=1
  Product : Product
  Saturation : Saturate  UpperLimit=(1*20)+1  LowerLimit=0
  Switch : Switch  Threshold=(1*20)  SaturateOnIntegerOverflow=off  InputSameDT=off
  and : Logic  AllPortsSameDT=off  OutDataTypeStr=boolean
  one : Constant
  zero : Constant  Value=0
  Fault_Out : Outport  VectorParamsAs1DForOutWhenUnconnected=off
  wires:
  and/1 -> Fault_Out/1
  Switch/1 -> and/1
  Delay1/1 -> Add/2
  one/1 -> Switch/1
  zero/1 -> Switch/3
  Add/1 -> Saturation/1
  Saturation/1 -> Product/2, Switch/2
  Product/1 -> Delay1/1
  Fault_In/1 -> and/2, Product/1, Add/1

== system SWC_AFE_Control/Subsystem/Debounce2 ==
  Fault_In : Inport
  Add : Sum
  Constant : Constant
  Delay1 : Delay  DelayLength=1
  Product : Product
  Saturation : Saturate  UpperLimit=(1*20)+1  LowerLimit=0
  Scope : Scope
  Switch : Switch  Threshold=(1*20)  SaturateOnIntegerOverflow=off  InputSameDT=off
  and : Logic  AllPortsSameDT=off  OutDataTypeStr=boolean
  one : Constant
  zero : Constant  Value=0
  Fault_Out : Outport  VectorParamsAs1DForOutWhenUnconnected=off
  wires:
  Constant/1 -> and/2, Add/1, Product/1
  Product/1 -> Delay1/1
  Saturation/1 -> Switch/2, Product/2
  Add/1 -> Saturation/1
  zero/1 -> Switch/3
  one/1 -> Switch/1
  Delay1/1 -> Add/2
  Switch/1 -> and/1
  and/1 -> Fault_Out/1

== system SWC_AFE_Control/Subsystem1/Debounce1 ==
  Fault_In : Inport
  Add : Sum
  Delay1 : Delay  DelayLength=1
  Product : Product
  Saturation : Saturate  UpperLimit=(0.1*1000)+1  LowerLimit=0
  Switch : Switch  Threshold=(0.1*1000)  SaturateOnIntegerOverflow=off  InputSameDT=off
  and : Logic  AllPortsSameDT=off  OutDataTypeStr=boolean
  one : Constant
  zero : Constant  Value=0
  Fault_Out : Outport  VectorParamsAs1DForOutWhenUnconnected=off
  wires:
  and/1 -> Fault_Out/1
  Switch/1 -> and/1
  Delay1/1 -> Add/2
  one/1 -> Switch/1
  zero/1 -> Switch/3
  Add/1 -> Saturation/1
  Saturation/1 -> Product/2, Switch/2
  Product/1 -> Delay1/1
  Fault_In/1 -> and/2, Product/1, Add/1

== system SWC_AFE_Control/Subsystem1/Debounce2 ==
  Fault_In : Inport
  Add : Sum
  Delay1 : Delay  DelayLength=1
  Product : Product
  Saturation : Saturate  UpperLimit=(0.1*1000)+1  LowerLimit=0
  Switch : Switch  Threshold=(0.1*1000)  SaturateOnIntegerOverflow=off  InputSameDT=off
  and : Logic  AllPortsSameDT=off  OutDataTypeStr=boolean
  one : Constant
  zero : Constant  Value=0
  Fault_Out : Outport  VectorParamsAs1DForOutWhenUnconnected=off
  wires:
  Fault_In/1 -> Add/1, Product/1, and/2
  Product/1 -> Delay1/1
  Saturation/1 -> Switch/2, Product/2
  Add/1 -> Saturation/1
  zero/1 -> Switch/3
  one/1 -> Switch/1
  Delay1/1 -> Add/2
  Switch/1 -> and/1
  and/1 -> Fault_Out/1

== system SWC_AFE_Control/Subsystem1/Debounce3 ==
  Fault_In : Inport
  Add : Sum
  Delay1 : Delay  DelayLength=1
  Product : Product
  Saturation : Saturate  UpperLimit=(0.1*1000)+1  LowerLimit=0
  Switch : Switch  Threshold=(0.1*1000)  SaturateOnIntegerOverflow=off  InputSameDT=off
  and : Logic  AllPortsSameDT=off  OutDataTypeStr=boolean
  one : Constant
  zero : Constant  Value=0
  Fault_Out : Outport  VectorParamsAs1DForOutWhenUnconnected=off
  wires:
  and/1 -> Fault_Out/1
  Switch/1 -> and/1
  Delay1/1 -> Add/2
  one/1 -> Switch/1
  zero/1 -> Switch/3
  Add/1 -> Saturation/1
  Saturation/1 -> Product/2, Switch/2
  Product/1 -> Delay1/1
  Fault_In/1 -> and/2, Product/1, Add/1

== system SWC_AFE_Control/Subsystem2/Debounce2 ==
  Fault_In : Inport
  Add : Sum
  Delay1 : Delay  DelayLength=1
  Product : Product
  Saturation : Saturate  UpperLimit=(40*0.24)+1  LowerLimit=0
  Switch : Switch  Threshold=(40*0.24)  SaturateOnIntegerOverflow=off  InputSameDT=off
  and : Logic  AllPortsSameDT=off  OutDataTypeStr=boolean
  one : Constant
  zero : Constant  Value=0
  Fault_Out : Outport  VectorParamsAs1DForOutWhenUnconnected=off
  wires:
  and/1 -> Fault_Out/1
  Switch/1 -> and/1
  Delay1/1 -> Add/2
  one/1 -> Switch/1
  zero/1 -> Switch/3
  Add/1 -> Saturation/1
  Saturation/1 -> Product/2, Switch/2
  Product/1 -> Delay1/1
  Fault_In/1 -> and/2, Product/1, Add/1

== system SWC_AFE_Control/Control_Loop/CONTROL/DCPICntrllr ==
  In2 : Inport
  In1 : Inport  Port=2
  In3 : Inport  Port=3
  In4 : Inport  Port=4
  In5 : Inport  Port=5
  In6 : Inport  Port=6
  In7 : Inport  Port=7
  In8 : Inport  Port=8
  Delay : Delay  DelayLength=1
  Delay1 : Delay  DelayLength=1
  Product{,1..3} (4 alike) : Product
  Saturation Dynamic : simulink/Discontinuities/Saturation Dynamic  OutMin=[]  OutMax=[]  OutDataTypeStr=Inherit: Same as second input  OutDataType=fixdt(1, 16)  OutScaling=2^-10  DoSatur=off
  Saturation Dynamic1 : simulink/Discontinuities/Saturation Dynamic  OutMin=[]  OutMax=[]  OutDataTypeStr=Inherit: Same as second input  OutDataType=fixdt(1, 16)  OutScaling=2^-10  DoSatur=off
  Saturation Dynamic2 : simulink/Discontinuities/Saturation Dynamic  OutMin=[]  OutMax=[]  OutDataTypeStr=Inherit: Same as second input  OutDataType=fixdt(1, 16)  OutScaling=2^-10  DoSatur=off
  Sum : Sum  Inputs=|+-
  Sum1 : Sum  Inputs=|++
  Sum2 : Sum  Inputs=|++
  Sum3 : Sum  Inputs=|+-
  Sum4 : Sum  Inputs=|-+
  Out1 : Outport
  wires:
  In2/1 -> Sum/2  "Act_rf"
  In1/1 -> Sum/1  "Ref_rf"
  Delay/1 -> Sum1/2  "Intgrl_Out_delay"
  Sum/1 -> Product1/1, Product/2
  In3/1 -> Product/1  "Kp_ff"
  Product/1 -> Saturation Dynamic/2
  In4/1 -> Product1/2  "Ki_ff"
  Product1/1 -> Delay1/1
  Delay1/1 -> Product2/1  "kierrgain"
  In5/1 -> Product2/2  "Ts_ff"
  Product2/1 -> Sum1/1
  Saturation Dynamic1/1 -> Product3/1
  In6/1 -> Product3/2  "Intgrl_reset_rb"
  Saturation Dynamic2/1 -> Out1/1  "Out"
  Sum1/1 -> Saturation Dynamic1/2
  In7/1 -> Sum3/1, Saturation Dynamic2/1, Saturation Dynamic/1  "ulim_ff"
  In8/1 -> Saturation Dynamic/3, Saturation Dynamic2/3, Sum4/2  "llimit_ff"
  Sum2/1 -> Saturation Dynamic2/2
  Product3/1 -> Delay/1, Sum2/2  "Intgrl_Out"
  Saturation Dynamic/1 -> Sum4/1, Sum3/2, Sum2/1  "Prpnl_Out"
  Sum4/1 -> Saturation Dynamic1/3
  Sum3/1 -> Saturation Dynamic1/1

== system SWC_AFE_Control/Control_Loop/CONTROL/Feed Forward ==
  In1 : Inport
  In2 : Inport  Port=2
  Input5 : Inport  Port=3
  Constant1 : Constant  Value=2*PI*INDUCTANCE  SampleTime=-1
  Product : Product
  Product1 : Product
  Product2 : Product
  Out1 : Outport
  Out2 : Outport  Port=2
  wires:
  In1/1 -> Product/1
  Product/1 -> Out2/1
  In2/1 -> Product1/2
  Product1/1 -> Out1/1
  Constant1/1 -> Product2/2
  Product2/1 -> Product1/1, Product/2
  Input5/1 -> Product2/1

== system SWC_AFE_Control/Control_Loop/CONTROL/IdPICntrllr ==
  In2 : Inport
  In1 : Inport  Port=2
  In3 : Inport  Port=3
  In4 : Inport  Port=4
  In5 : Inport  Port=5
  In6 : Inport  Port=6
  In7 : Inport  Port=7
  In8 : Inport  Port=8
  Delay : Delay  DelayLength=1
  Delay1 : Delay  DelayLength=1
  Product{,1..3} (4 alike) : Product
  Saturation Dynamic : simulink/Discontinuities/Saturation Dynamic  OutMin=[]  OutMax=[]  OutDataTypeStr=Inherit: Same as second input  OutDataType=fixdt(1, 16)  OutScaling=2^-10  DoSatur=off
  Saturation Dynamic1 : simulink/Discontinuities/Saturation Dynamic  OutMin=[]  OutMax=[]  OutDataTypeStr=Inherit: Same as second input  OutDataType=fixdt(1, 16)  OutScaling=2^-10  DoSatur=off
  Saturation Dynamic2 : simulink/Discontinuities/Saturation Dynamic  OutMin=[]  OutMax=[]  OutDataTypeStr=Inherit: Same as second input  OutDataType=fixdt(1, 16)  OutScaling=2^-10  DoSatur=off
  Sum : Sum  Inputs=|+-
  Sum1 : Sum  Inputs=|++  OutDataTypeStr=single
  Sum2 : Sum  Inputs=|++  OutDataTypeStr=single
  Sum3 : Sum  Inputs=|+-
  Sum4 : Sum  Inputs=|-+
  Out1 : Outport
  wires:
  In2/1 -> Sum/2  "Act_rf"
  In1/1 -> Sum/1  "Ref_rf"
  Delay/1 -> Sum1/2  "Intgrl_Out_delay"
  Sum/1 -> Product1/1, Product/2
  In3/1 -> Product/1  "Kp_ff"
  Product/1 -> Saturation Dynamic/2
  In4/1 -> Product1/2  "Ki_ff"
  Product1/1 -> Delay1/1
  Delay1/1 -> Product2/1  "kierrgain"
  In5/1 -> Product2/2  "Ts_ff"
  Product2/1 -> Sum1/1
  Saturation Dynamic1/1 -> Product3/1
  In6/1 -> Product3/2  "Intgrl_reset_rb"
  Saturation Dynamic2/1 -> Out1/1  "Out"
  Sum1/1 -> Saturation Dynamic1/2
  In7/1 -> Sum3/1, Saturation Dynamic2/1, Saturation Dynamic/1  "ulim_ff"
  In8/1 -> Saturation Dynamic/3, Saturation Dynamic2/3, Sum4/2  "llimit_ff"
  Sum2/1 -> Saturation Dynamic2/2
  Product3/1 -> Delay/1, Sum2/2  "Intgrl_Out"
  Saturation Dynamic/1 -> Sum4/1, Sum3/2, Sum2/1  "Prpnl_Out"
  Sum4/1 -> Saturation Dynamic1/3
  Sum3/1 -> Saturation Dynamic1/1

== system SWC_AFE_Control/Control_Loop/CONTROL/IqPICntrllr ==
  In2 : Inport
  In1 : Inport  Port=2
  In3 : Inport  Port=3
  In4 : Inport  Port=4
  In5 : Inport  Port=5
  In6 : Inport  Port=6
  In7 : Inport  Port=7
  In8 : Inport  Port=8
  Delay : Delay  DelayLength=1
  Delay1 : Delay  DelayLength=1
  Product{,1..3} (4 alike) : Product
  Saturation Dynamic : simulink/Discontinuities/Saturation Dynamic  OutMin=[]  OutMax=[]  OutDataTypeStr=Inherit: Same as second input  OutDataType=fixdt(1, 16)  OutScaling=2^-10  DoSatur=off
  Saturation Dynamic1 : simulink/Discontinuities/Saturation Dynamic  OutMin=[]  OutMax=[]  OutDataTypeStr=Inherit: Same as second input  OutDataType=fixdt(1, 16)  OutScaling=2^-10  DoSatur=off
  Saturation Dynamic2 : simulink/Discontinuities/Saturation Dynamic  OutMin=[]  OutMax=[]  OutDataTypeStr=Inherit: Same as second input  OutDataType=fixdt(1, 16)  OutScaling=2^-10  DoSatur=off
  Sum : Sum  Inputs=|+-
  Sum1 : Sum  Inputs=|++  OutDataTypeStr=single
  Sum2 : Sum  Inputs=|++  OutDataTypeStr=single
  Sum3 : Sum  Inputs=|+-
  Sum4 : Sum  Inputs=|-+
  Out1 : Outport
  wires:
  In2/1 -> Sum/2  "Act_rf"
  In1/1 -> Sum/1  "Ref_rf"
  Delay/1 -> Sum1/2  "Intgrl_Out_delay"
  Sum/1 -> Product1/1, Product/2
  In3/1 -> Product/1  "Kp_ff"
  Product/1 -> Saturation Dynamic/2
  In4/1 -> Product1/2  "Ki_ff"
  Product1/1 -> Delay1/1
  Delay1/1 -> Product2/1  "kierrgain"
  In5/1 -> Product2/2  "Ts_ff"
  Product2/1 -> Sum1/1
  Saturation Dynamic1/1 -> Product3/1
  In6/1 -> Product3/2  "Intgrl_reset_rb"
  Saturation Dynamic2/1 -> Out1/1  "Out"
  Sum1/1 -> Saturation Dynamic1/2
  In7/1 -> Sum3/1, Saturation Dynamic2/1, Saturation Dynamic/1  "ulim_ff"
  In8/1 -> Saturation Dynamic/3, Saturation Dynamic2/3, Sum4/2  "llimit_ff"
  Sum2/1 -> Saturation Dynamic2/2
  Product3/1 -> Delay/1, Sum2/2  "Intgrl_Out"
  Saturation Dynamic/1 -> Sum4/1, Sum3/2, Sum2/1  "Prpnl_Out"
  Sum4/1 -> Saturation Dynamic1/3
  Sum3/1 -> Saturation Dynamic1/1

== system SWC_AFE_Control/Control_Loop/CONTROL/abctodq ==
  ph_a : Inport
  ph_b : Inport  Port=2
  ph_c : Inport  Port=3
  sinthetha : Inport  Port=4
  costhetha : Inport  Port=5
  abctoalphabeta : Subsystem
  alphabetatodq : Subsystem
  alpha : Outport
  beta : Outport  Port=2
  d : Outport  Port=3
  q : Outport  Port=4
  wires:
  sinthetha/1 -> alphabetatodq/3(sinthetha)  "sinthetha"
  costhetha/1 -> alphabetatodq/4(costhetha)  "costhetha"
  ph_a/1 -> abctoalphabeta/1(ph_a)  "ph_a"
  ph_b/1 -> abctoalphabeta/2(ph_b)  "ph_b"
  ph_c/1 -> abctoalphabeta/3(ph_c)  "ph_c"
  abctoalphabeta/2(beta) -> alphabetatodq/2(beta), beta/1  "beta"
  abctoalphabeta/1(alpha) -> alpha/1, alphabetatodq/1(alpha)  "alpha"
  alphabetatodq/2(q) -> q/1  "q"
  alphabetatodq/1(d) -> d/1  "d"

== system SWC_AFE_Control/Control_Loop/CONTROL/dqtoabc ==
  ref_d : Inport
  ref_q : Inport  Port=2
  ref_sinthetha : Inport  Port=3
  ref_costhetha : Inport  Port=4
  alphabetatoabc : Subsystem
  dqtoalphabeta : Subsystem
  ref_alpha : Outport
  ref_beta : Outport  Port=2
  ph_a : Outport  Port=3
  ph_b : Outport  Port=4
  ph_c : Outport  Port=5
  wires:
  ref_sinthetha/1 -> dqtoalphabeta/3(Input1)  "ref_sinthetha"
  ref_costhetha/1 -> dqtoalphabeta/4(Input)  "ref_costhetha"
  dqtoalphabeta/1(alpha) -> alphabetatoabc/1(Input), ref_alpha/1  "ref_alpha"
  dqtoalphabeta/2(beta) -> alphabetatoabc/2(Input1), ref_beta/1  "ref_beta"
  ref_d/1 -> dqtoalphabeta/1(Input2)  "ref_d"
  ref_q/1 -> dqtoalphabeta/2(Input3)  "ref_q"
  alphabetatoabc/1(ph_a) -> ph_a/1  "ref_ph_a"
  alphabetatoabc/2(ph_b) -> ph_b/1  "ref_ph_b"
  alphabetatoabc/3(ph_c) -> ph_c/1  "ref_ph_c"

== system SWC_AFE_Control/PWM_Loop/Fault/CurrentFaults ==
  Ia_adc_ru2 : Inport
  Ib_adc_ru2 : Inport  Port=2
  Ic_adc_ru2 : Inport  Port=3
  Iabc_offset_ru2 : Inport  Port=4
  AFE_State_ID : Inport  Port=5
  PhA_CurrSnsr_Fault : Subsystem  TreatAsAtomicUnit=on
      settings: RTWFcnNameOpts=Use subsystem name  RTWFileNameOpts=Use subsystem name
  PhB_CurrSnsr_Fault : Subsystem  TreatAsAtomicUnit=on
  PhC_CurrSnsr_Fault : Subsystem  TreatAsAtomicUnit=on
  Out1 : Outport
  Out2 : Outport  Port=2
  Out3 : Outport  Port=3
  wires:
  Ia_adc_ru2/1 -> PhA_CurrSnsr_Fault/1(In1)
  Iabc_offset_ru2/1 -> PhC_CurrSnsr_Fault/2(Iabc_offset_ru2), PhB_CurrSnsr_Fault/2(Iabc_offset_ru2), PhA_CurrSnsr_Fault/2(In2)
  AFE_State_ID/1 -> PhC_CurrSnsr_Fault/3(AFE_State_ID), PhB_CurrSnsr_Fault/3(AFE_State_ID), PhA_CurrSnsr_Fault/3(In3)
  PhA_CurrSnsr_Fault/1(Out1) -> Out1/1  "AFE_PhA_CurrSnsr_Fault_st_enum"
  PhC_CurrSnsr_Fault/1(Out1) -> Out3/1  "AFE_PhC_CurrSnsr_Fault_st_enum"
  Ic_adc_ru2/1 -> PhC_CurrSnsr_Fault/1(Ic_adc_ru2)
  Ib_adc_ru2/1 -> PhB_CurrSnsr_Fault/1(Ib_adc_ru2)
  PhB_CurrSnsr_Fault/1(Out1) -> Out2/1  "AFE_PhB_CurrSnsr_Fault_st_enum"

== system SWC_AFE_Control/PWM_Loop/PLL/Integrator ==
  Omega : Inport
  Add : Sum
  Constant1 : Constant  Value=PI  OutDataTypeStr=single
  Data Type Conversion : DataTypeConversion  OutDataTypeStr=single  SaturateOnIntegerOverflow=off  RndMeth=Floor
  INTEGRATOR_WRAP : Scope
  INTEGRATOR_WRAP1 : Scope
  Kp1 : Gain  Gain=PLL_RATE  SaturateOnIntegerOverflow=on  OutDataTypeStr=Inherit: Same as input  ParamDataTypeStr=Inherit: Same as input
  Mux3 : Mux  Inputs=3
  Unit Delay1 : UnitDelay  InitialCondition=2*pi*50  SampleTime=-1  HasFrameUpgradeWarning=on
  WrapRange : Subsystem
  Angle : Outport  InitialOutput=0
  wires:
  Kp1/1 -> INTEGRATOR_WRAP1/1, Add/1
  Omega/1 -> Kp1/1
  Unit Delay1/1 -> Add/2, Mux3/1
  Constant1/1 -> WrapRange/2(range)
  Mux3/1 -> INTEGRATOR_WRAP/1
  WrapRange/1(WRAP_ANGLE) -> Data Type Conversion/1, Unit Delay1/1, Mux3/3
  Add/1 -> WrapRange/1(Omega_1), Mux3/2
  Data Type Conversion/1 -> Angle/1
